simulink model "Q2_Pendulum_Osicllator"  (R2024b)
settings: Solver=VariableStepAuto  StartTime=0.0  StopTime=15  RelTol=1e-3
model workspace (MAT data in the model file):
  I_0 = 0.008
  I_o = 0.088
  L = 0.43
  g = 9.81
  m = 1
settings Model: Creator=chall  LastModifiedBy=chall

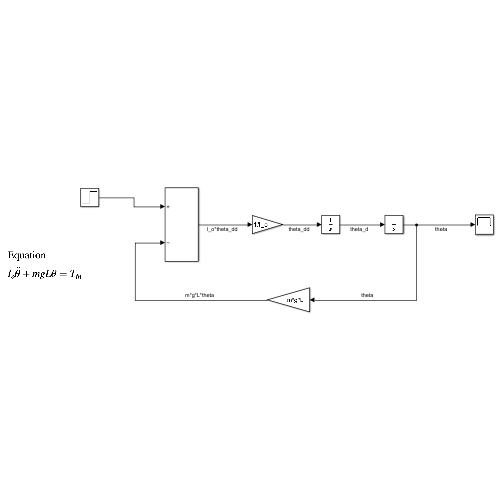
[thumbnail: Simulink's stored preview of the top-level diagram]
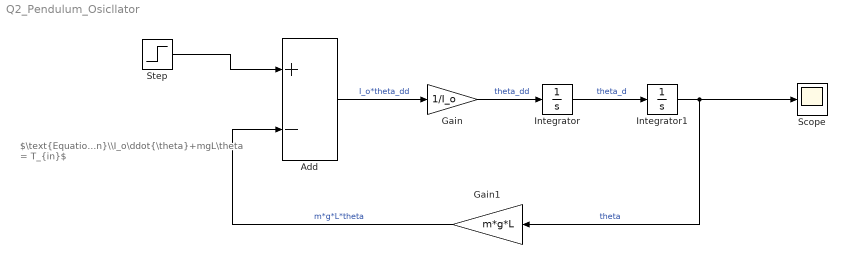
== system Q2_Pendulum_Osicllator ==
  note: $\text{Equation}\\I_o\ddot{\theta}+mgL\theta = T_{in}$
  Add : Sum  Inputs=+-
  Gain : Gain  Gain=1/I_o
  Gain1 : Gain  Gain=m*g*L
  Integrator : Integrator
  Integrator1 : Integrator
  Scope : Scope
  Step : Step  Time=0  SampleTime=0
  wires:
  Add/1 -> Gain/1  "I_o*theta_dd"
  Gain/1 -> Integrator/1  "theta_dd"
  Integrator/1 -> Integrator1/1  "theta_d"
  Integrator1/1 -> Gain1/1, Scope/1  "theta"
  Gain1/1 -> Add/2  "m*g*L*theta"
  Step/1 -> Add/1
